simulink model "eg5p3"  (Simulink 2.09)
settings: Solver=ode45  StartTime=0.0  StopTime=20.0  RelTol=1e-3  AbsTol=1e-6
settings Model: ConsistencyChecking=off  RTWTemplateMakefile=grt_unix.tmf

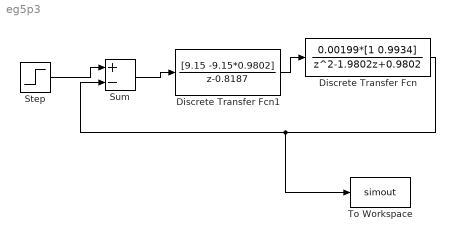
== system eg5p3 ==
  Discrete Transfer Fcn : DiscreteTransferFcn  Numerator=0.00199*[1 0.9934]  Denominator=[1 -1.9802 0.9802]  SampleTime=0.2
  Discrete Transfer Fcn1 : DiscreteTransferFcn  Numerator=[9.15 -9.15*0.9802]  Denominator=[1 -0.8187]  SampleTime=0.2
  Step : Step  Time=1  Before=0  After=1
  Sum : Sum  Inputs=+-
  To Workspace : ToWorkspace  VariableName=simout  SampleTime=-1
  wires:
  Discrete Transfer Fcn/1 -> To Workspace/1, Sum/2
  Step/1 -> Sum/1
  Discrete Transfer Fcn1/1 -> Discrete Transfer Fcn/1
  Sum/1 -> Discrete Transfer Fcn1/1
